simulink model "RizzoRezEq2"  (Simulink 7.2)
settings: Solver=ode45  StartTime=0.0  StopTime=10.0  MaxStep=0.000001  RelTol=1e-3
values from neighbouring files (symbols this model uses):
  Bc = 0    [TFconfirm.m]    (also in Torsonal_Model_Constants.m = 0.01)
  Ja = Ja+JL    (= 0.0056)    [TFconfirm.m]
  JL = 0.0033    [TFconfirm.m]    (also in Torsonal_Model_Constants.m)
  Ka = 10    [PlotRizzo.m]    (also in RizzoRezEqBode.m; TFconfirm.m)
  Kc = 0    [TFconfirm.m]
  Ke = 0.042685    [PlotRizzo.m]    (also in RizzoRezEqBode.m; TFconfirm.m)
  ki = 0.2    [PlotRizzo.m]    (also in RizzoRezEqBode.m = 0.02; TFconfirm.m)
  Kt = 6.046    [PlotRizzo.m]    (also in RizzoRezEqBode.m; TFconfirm.m)
  kv = 20    [PlotRizzo.m]    (also in RizzoRezEqBode.m; TFconfirm.m)
  L = 0.842    [PlotRizzo.m]    (also in RizzoRezEqBode.m; TFconfirm.m)
  Ra = 0.38    [PlotRizzo.m]    (also in RizzoRezEqBode.m; TFconfirm.m)
settings Model: Creator=geovana  LastModifiedBy=geovana
settings DebuggingCC: StrictBusMsg=ErrorLevel1

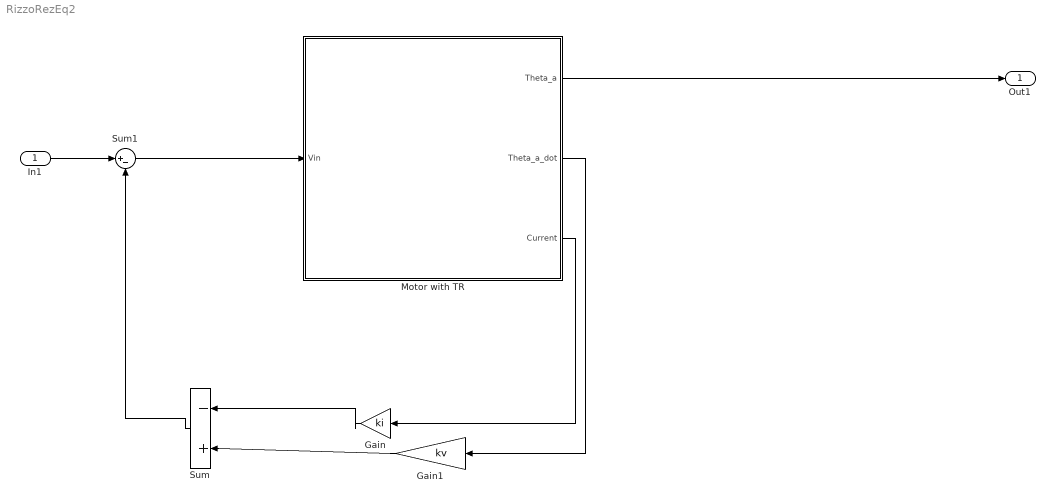
== system RizzoRezEq2 ==
  In1 : Inport  OutDataType=fixdt(1, 16)  OutScaling=2^0
  Gain : Gain  Orientation=left  Gain=ki  ParameterDataType=fixdt(1, 16)  ParameterScaling=2^0  OutDataType=fixdt(1, 16)  OutScaling=2^0
  Gain1 : Gain  Orientation=left  Gain=kv  ParameterDataType=fixdt(1, 16)  ParameterScaling=2^0  OutDataType=fixdt(1, 16)  OutScaling=2^0
  Motor with TR : Subsystem
  Sum : Sum  Orientation=left  Inputs=|-+  OutDataType=fixdt(1, 16)  OutScaling=2^0
  Sum1 : Sum  Inputs=|+-  OutDataType=fixdt(1, 16)  OutScaling=2^0
  Out1 : Outport  OutDataType=fixdt(1, 16)  OutScaling=2^0
  wires:
  Motor with TR/1(Theta_a) -> Out1/1
  In1/1 -> Sum1/1
  Sum1/1 -> Motor with TR/1(Vin)
  Sum/1 -> Sum1/2
  Gain1/1 -> Sum/2
  Gain/1 -> Sum/1
  Motor with TR/3(Current) -> Gain/1
  Motor with TR/2(Theta_a_dot) -> Gain1/1

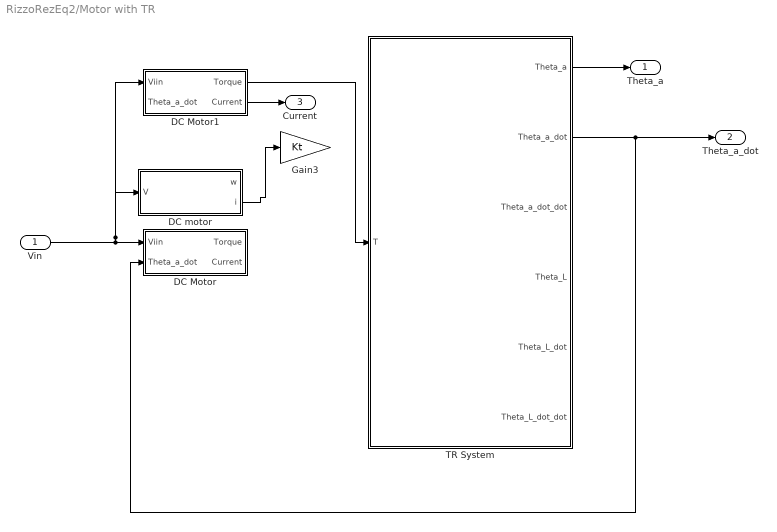
== system RizzoRezEq2/Motor with TR ==
  Vin : Inport  OutDataType=fixdt(1, 16)  OutScaling=2^0
  DC Motor : Subsystem
  DC Motor1 : Subsystem
  DC motor : Subsystem  mask(DC Motor){L=0.1, Kphi=0.3, J=0.1, b=0.01, R=2}
      mask help:
      | Takes the DC voltage as input, and outputs angular velocity (w) and current (i)
      | L => windings inductance		Kphi => emf constant
      | J => loads moment of inertial		b => viscous friction
      | R => windings resistance
      mask Display:
      | port_label('input', 1, 'V')
      | port_label('output', 2, 'i')
      | port_label('output', 1, 'w')
      | disp('DC Motor')
  Gain3 : Gain  Gain=Kt  ParameterDataType=fixdt(1, 16)  ParameterScaling=2^0  OutDataType=fixdt(1, 16)  OutScaling=2^0
  TR System : Subsystem
  Theta_a : Outport  OutDataType=fixdt(1, 16)  OutScaling=2^0
  Theta_a_dot : Outport  Port=2  OutDataType=fixdt(1, 16)  OutScaling=2^0
  Current : Outport  Port=3
  wires:
  TR System/2(Theta_a_dot) -> DC Motor/2(Theta_a_dot), Theta_a_dot/1
  Vin/1 -> DC Motor/1(Viin), DC motor/1(V), DC Motor1/1(Viin)
  TR System/1(Theta_a) -> Theta_a/1
  DC motor/2(i) -> Gain3/1
  DC Motor1/1(Torque) -> TR System/1(T)
  DC Motor1/2(Current) -> Current/1

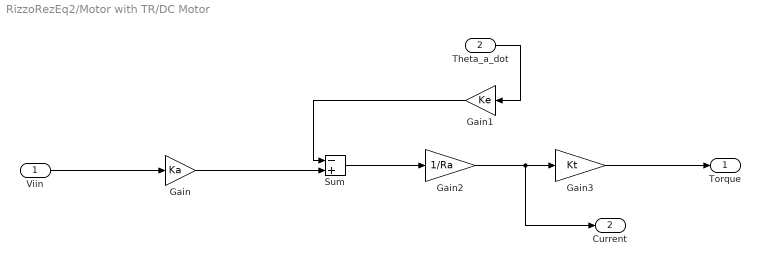
== system RizzoRezEq2/Motor with TR/DC Motor ==
  Viin : Inport  OutDataType=fixdt(1, 16)  OutScaling=2^0
  Theta_a_dot : Inport  Port=2  OutDataType=fixdt(1, 16)  OutScaling=2^0
  Gain : Gain  Gain=Ka  ParameterDataType=fixdt(1, 16)  ParameterScaling=2^0  OutDataType=fixdt(1, 16)  OutScaling=2^0
  Gain1 : Gain  Orientation=left  Gain=Ke  ParameterDataType=fixdt(1, 16)  ParameterScaling=2^0  OutDataType=fixdt(1, 16)  OutScaling=2^0
  Gain2 : Gain  Gain=1/Ra  ParameterDataType=fixdt(1, 16)  ParameterScaling=2^0  OutDataType=fixdt(1, 16)  OutScaling=2^0
  Gain3 : Gain  Gain=Kt  ParameterDataType=fixdt(1, 16)  ParameterScaling=2^0  OutDataType=fixdt(1, 16)  OutScaling=2^0
  Sum : Sum  Inputs=|-+  OutDataType=fixdt(1, 16)  OutScaling=2^0
  Torque : Outport  OutDataType=fixdt(1, 16)  OutScaling=2^0
  Current : Outport  Port=2  OutDataType=fixdt(1, 16)  OutScaling=2^0
  wires:
  Viin/1 -> Gain/1
  Gain/1 -> Sum/2
  Sum/1 -> Gain2/1
  Gain2/1 -> Gain3/1, Current/1
  Gain3/1 -> Torque/1
  Theta_a_dot/1 -> Gain1/1
  Gain1/1 -> Sum/1

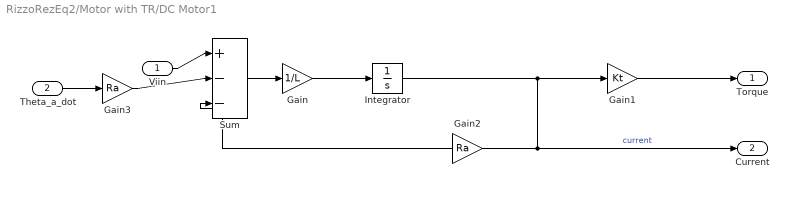
== system RizzoRezEq2/Motor with TR/DC Motor1 ==
  Viin : Inport  OutDataType=fixdt(1, 16)  OutScaling=2^0
  Theta_a_dot : Inport  Port=2  OutDataType=fixdt(1, 16)  OutScaling=2^0
  Gain : Gain  Gain=1/L  ParameterDataType=fixdt(1, 16)  ParameterScaling=2^0  OutDataType=fixdt(1, 16)  OutScaling=2^0
  Gain1 : Gain  Gain=Kt  ParameterDataType=fixdt(1, 16)  ParameterScaling=2^0  OutDataType=fixdt(1, 16)  OutScaling=2^0
  Gain2 : Gain  Gain=Ra  ParameterDataType=fixdt(1, 16)  ParameterScaling=2^0  OutDataType=fixdt(1, 16)  OutScaling=2^0
  Gain3 : Gain  Gain=Ra  ParameterDataType=fixdt(1, 16)  ParameterScaling=2^0  OutDataType=fixdt(1, 16)  OutScaling=2^0
  Integrator : Integrator
  Sum : Sum  Inputs=|+--  OutDataType=fixdt(1, 16)  OutScaling=2^0
  Torque : Outport  OutDataType=fixdt(1, 16)  OutScaling=2^0
  Current : Outport  Port=2  OutDataType=fixdt(1, 16)  OutScaling=2^0
  wires:
  Viin/1 -> Sum/1
  Sum/1 -> Gain/1
  Gain/1 -> Integrator/1
  Integrator/1 -> Gain1/1, Current/1, Gain2/1  "current"
  Gain1/1 -> Torque/1
  Gain2/1 -> Sum/3
  Theta_a_dot/1 -> Gain3/1
  Gain3/1 -> Sum/2

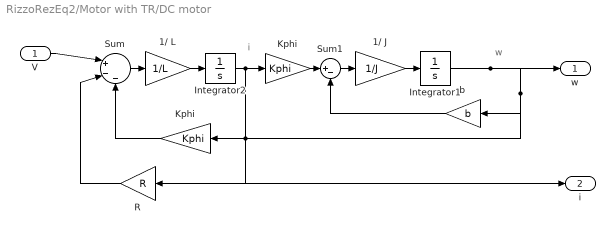
== system RizzoRezEq2/Motor with TR/DC motor ==
  note: i
  note: w
  V : Inport  OutDataType=sfix(16)  OutScaling=2^0
  1/ J : Gain  Gain=1/J  ParameterDataType=sfix(16)  ParameterScaling=2^0  OutDataType=sfix(16)  OutScaling=2^0
  1/ L : Gain  Gain=1/L  ParameterDataType=sfix(16)  ParameterScaling=2^0  OutDataType=sfix(16)  OutScaling=2^0
  Integrator1 : Integrator
  Integrator2 : Integrator
  Kphi : Gain  Gain=Kphi  ParameterDataType=sfix(16)  ParameterScaling=2^0  OutDataType=sfix(16)  OutScaling=2^0
  "Kphi " : Gain  Orientation=left  Gain=Kphi  ParameterDataType=sfix(16)  ParameterScaling=2^0  OutDataType=sfix(16)  OutScaling=2^0
  R : Gain  Orientation=left  Gain=R  ParameterDataType=sfix(16)  ParameterScaling=2^0  OutDataType=sfix(16)  OutScaling=2^0
  Sum : Sum  Inputs=|+--  OutDataType=sfix(16)  OutScaling=2^0
  Sum1 : Sum  Inputs=|+-  OutDataType=sfix(16)  OutScaling=2^0
  b : Gain  Orientation=left  Gain=b  ParameterDataType=sfix(16)  ParameterScaling=2^0  OutDataType=sfix(16)  OutScaling=2^0
  w : Outport  OutDataType=sfix(16)  OutScaling=2^0
  i : Outport  Port=2  OutDataType=sfix(16)  OutScaling=2^0
  wires:
  V/1 -> Sum/1
  Sum/1 -> 1/ L/1
  1/ L/1 -> Integrator2/1
  Integrator2/1 -> Kphi/1, R/1, i/1
  Kphi/1 -> Sum1/1
  Sum1/1 -> 1/ J/1
  1/ J/1 -> Integrator1/1
  Integrator1/1 -> "Kphi "/1, b/1, w/1
  b/1 -> Sum1/2
  "Kphi "/1 -> Sum/3
  R/1 -> Sum/2

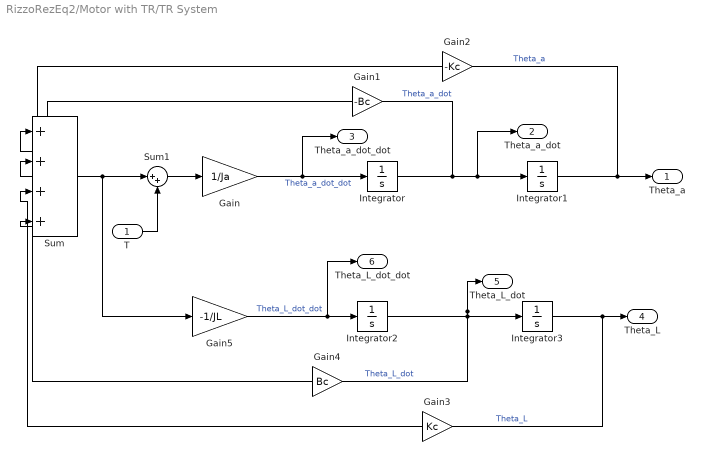
== system RizzoRezEq2/Motor with TR/TR System ==
  T : Inport  OutDataType=sfix(16)  OutScaling=2^0
  Gain : Gain  Gain=1/Ja  ParameterDataType=sfix(16)  ParameterScaling=2^0  OutDataType=sfix(16)  OutScaling=2^0
  Gain1 : Gain  Gain=-Bc  ParameterDataType=sfix(16)  ParameterScaling=2^0  OutDataType=sfix(16)  OutScaling=2^0
  Gain2 : Gain  Gain=-Kc  ParameterDataType=sfix(16)  ParameterScaling=2^0  OutDataType=sfix(16)  OutScaling=2^0
  Gain3 : Gain  Gain=Kc  ParameterDataType=sfix(16)  ParameterScaling=2^0  OutDataType=sfix(16)  OutScaling=2^0
  Gain4 : Gain  Gain=Bc  ParameterDataType=sfix(16)  ParameterScaling=2^0  OutDataType=sfix(16)  OutScaling=2^0
  Gain5 : Gain  Gain=-1/JL  ParameterDataType=sfix(16)  ParameterScaling=2^0  OutDataType=sfix(16)  OutScaling=2^0
  Integrator{,1..3} (4 alike) : Integrator
  Sum : Sum  Inputs=|++++  OutDataType=sfix(16)  OutScaling=2^0
  Sum1 : Sum  Inputs=|++  OutDataType=sfix(16)  OutScaling=2^0
  Theta_a : Outport  OutDataType=sfix(16)  OutScaling=2^0
  Theta_a_dot : Outport  Port=2  OutDataType=sfix(16)  OutScaling=2^0
  Theta_a_dot_dot : Outport  Port=3  OutDataType=sfix(16)  OutScaling=2^0
  Theta_L : Outport  Port=4  OutDataType=sfix(16)  OutScaling=2^0
  Theta_L_dot : Outport  Port=5  OutDataType=sfix(16)  OutScaling=2^0
  Theta_L_dot_dot : Outport  Port=6  OutDataType=sfix(16)  OutScaling=2^0
  wires:
  Sum/1 -> Gain5/1, Sum1/1
  Integrator/1 -> Gain1/1, Integrator1/1, Theta_a_dot/1  "Theta_a_dot"
  Integrator1/1 -> Gain2/1, Theta_a/1  "Theta_a"
  Gain1/1 -> Sum/1
  Gain2/1 -> Sum/2
  Gain/1 -> Integrator/1, Theta_a_dot_dot/1  "Theta_a_dot_dot"
  Integrator2/1 -> Integrator3/1, Gain4/1, Theta_L_dot/1  "Theta_L_dot"
  Gain5/1 -> Integrator2/1, Theta_L_dot_dot/1  "Theta_L_dot_dot"
  Sum1/1 -> Gain/1
  T/1 -> Sum1/2
  Integrator3/1 -> Theta_L/1, Gain3/1  "Theta_L"
  Gain3/1 -> Sum/3
  Gain4/1 -> Sum/4
